simulink model "FAST_Model"  (R2020a)
settings: Solver=FixedStepAuto  StartTime=0.0  StopTime=10.0  FixedStep=DT  RelTol=1e-3
values from neighbouring files (symbols this model uses):
  g = 97    [run_Top_Model.m]    (also in turbine_params_5MW.m = @(theta) f(tp.v_x_bp(k),theta))
  OutList = get_OutList(outfile_path)    [run_Top_Model_multi.m]
undefined symbols (not defined in the file or in its folder): strmatch
settings Model: Creator=lpwoolcock  LastModifiedBy=lpwoolcock

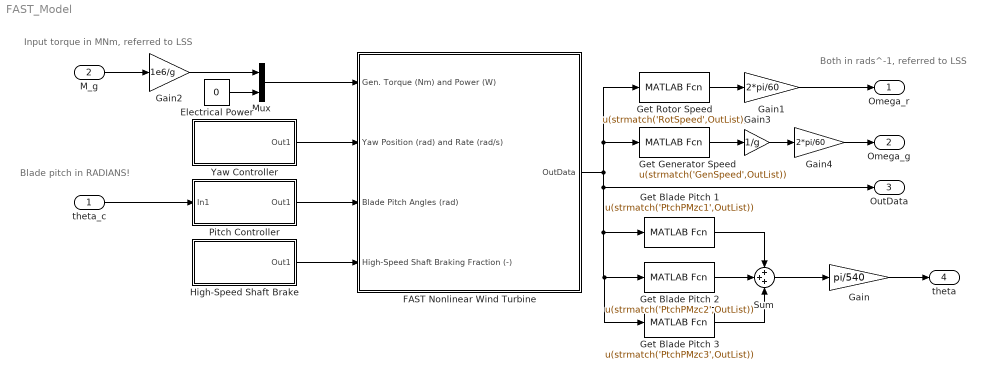
== system FAST_Model ==
  note: Input torque in MNm, referred to LSS
  note: Both in rads^-1, referred to LSS
  note: Blade pitch in RADIANS!
  theta_c : Inport
  M_g : Inport  Port=2
  Electrical Power : Constant  Value=0
  FAST Nonlinear Wind Turbine : Subsystem  mask(FAST Nonlinear Wind Turbine){}
      mask help: This block contains the FAST S-Function.
      mask init:
      | clear FAST_SFunc
  Gain : Gain  Gain=pi/540
  Gain1 : Gain  Gain=2*pi/60
  Gain2 : Gain  Gain=1e6/g
  Gain3 : Gain  Gain=1/g
  Gain4 : Gain  Gain=2*pi/60
  Get Blade Pitch 1 : MATLABFcn  MATLABFcn=u(strmatch('PtchPMzc1',OutList))
  Get Blade Pitch 2 : MATLABFcn  MATLABFcn=u(strmatch('PtchPMzc2',OutList))
  Get Blade Pitch 3 : MATLABFcn  MATLABFcn=u(strmatch('PtchPMzc3',OutList))
  Get Generator Speed : MATLABFcn  MATLABFcn=u(strmatch('GenSpeed',OutList))
  Get Rotor Speed : MATLABFcn  MATLABFcn=u(strmatch('RotSpeed',OutList))
  High-Speed Shaft Brake : Subsystem
  Mux : Mux  Inputs=2
  Pitch Controller : Subsystem
  Sum : Sum  Inputs=+++
  Yaw Controller : Subsystem
  Omega_r : Outport
  Omega_g : Outport  Port=2
  OutData : Outport  Port=3
  theta : Outport  Port=4
  wires:
  Gain2/1 -> Mux/1
  Yaw Controller/1(Out1) -> FAST Nonlinear Wind Turbine/2(Yaw Position (rad) and Rate (rad/s))
  Get Rotor Speed/1 -> Gain1/1
  Mux/1 -> FAST Nonlinear Wind Turbine/1(Gen. Torque (Nm) and Power (W))
  High-Speed Shaft Brake/1(Out1) -> FAST Nonlinear Wind Turbine/4(High-Speed Shaft Braking Fraction (-))
  Electrical Power/1 -> Mux/2
  FAST Nonlinear Wind Turbine/1(OutData) -> Get Blade Pitch 3/1, Get Blade Pitch 2/1, Get Blade Pitch 1/1, OutData/1, Get Generator Speed/1, Get Rotor Speed/1
  Gain1/1 -> Omega_r/1
  Pitch Controller/1(Out1) -> FAST Nonlinear Wind Turbine/3(Blade Pitch Angles (rad))
  Gain3/1 -> Gain4/1
  theta_c/1 -> Pitch Controller/1(In1)
  Get Generator Speed/1 -> Gain3/1
  M_g/1 -> Gain2/1
  Gain4/1 -> Omega_g/1
  Sum/1 -> Gain/1
  Get Blade Pitch 2/1 -> Sum/2
  Get Blade Pitch 1/1 -> Sum/1
  Get Blade Pitch 3/1 -> Sum/3
  Gain/1 -> theta/1

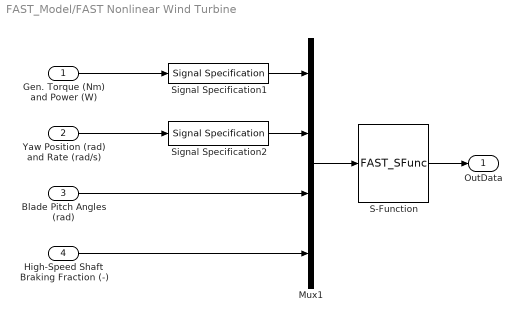
== system FAST_Model/FAST Nonlinear Wind Turbine ==
  Gen. Torque (Nm) and Power (W) : Inport
  Yaw Position (rad) and Rate (rad/s) : Inport  Port=2
  Blade Pitch Angles (rad) : Inport  Port=3
  High-Speed Shaft Braking Fraction (-) : Inport  Port=4
  Mux1 : Mux
  S-Function : S-Function  FunctionName=FAST_SFunc  Parameters=FAST_InputFileName, TMax, 0  SFunctionDeploymentMode=off  EnableBusSupport=off
  Signal Specification1 : SignalSpecification  OutDataTypeStr=double  Dimensions=2
  Signal Specification2 : SignalSpecification  OutDataTypeStr=double  Dimensions=2
  OutData : Outport  VectorParamsAs1DForOutWhenUnconnected=off
  wires:
  Gen. Torque (Nm) and Power (W)/1 -> Signal Specification1/1
  S-Function/1 -> OutData/1
  Mux1/1 -> S-Function/1
  Blade Pitch Angles (rad)/1 -> Mux1/3
  Yaw Position (rad) and Rate (rad/s)/1 -> Signal Specification2/1
  Signal Specification1/1 -> Mux1/1
  Signal Specification2/1 -> Mux1/2
  High-Speed Shaft Braking Fraction (-)/1 -> Mux1/4

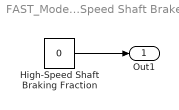
== system FAST_Model/High-Speed Shaft Brake ==
  High-Speed Shaft Braking Fraction : Constant  Value=0
  Out1 : Outport  VectorParamsAs1DForOutWhenUnconnected=off
  wires:
  High-Speed Shaft Braking Fraction/1 -> Out1/1

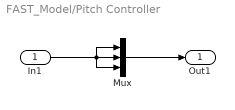
== system FAST_Model/Pitch Controller ==
  In1 : Inport
  Mux : Mux  Inputs=3
  Out1 : Outport  VectorParamsAs1DForOutWhenUnconnected=off
  wires:
  Mux/1 -> Out1/1
  In1/1 -> Mux/3, Mux/2, Mux/1

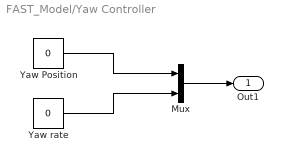
== system FAST_Model/Yaw Controller ==
  Mux : Mux  Inputs=2
  Yaw Position : Constant  Value=0
  Yaw rate : Constant  Value=0
  Out1 : Outport  VectorParamsAs1DForOutWhenUnconnected=off
  wires:
  Mux/1 -> Out1/1
  Yaw Position/1 -> Mux/1
  Yaw rate/1 -> Mux/2
